simulink library "MISSILE_GUIDANCE_LIB2"  (R2025b)
settings: Solver=VariableStepAuto  StartTime=0.0  StopTime=10.0  RelTol=1e-3
undefined symbols (not defined in the file or in its folder): accelerationL0, angularPoseL0, angularRateL0, B2D, Continuous, ddLambda, dLambda, dRange, epsMEAS_D, L02B, Lambda, positionL0, psiDotCmd, psiMeas, Range, rangeDotMEAS_D, rangeMEAS_D, t_go, t_sim, targetEps_D, targetRelPos_B, targetRelPos_D, targetRelPos_L0, targetRelVel_L0, targetValid, thetaDotCmd, thetaMeas, Time, timeOfMeas, velocityL0, wAfterStabTF, wCmd_Rtn
libraries: $bdroot x27, simulink x8, simulink_extras x6, matrix_library x3, Missile_Guidance_LIB x1, ctrlSharedLib x1
(part 2 of 2)

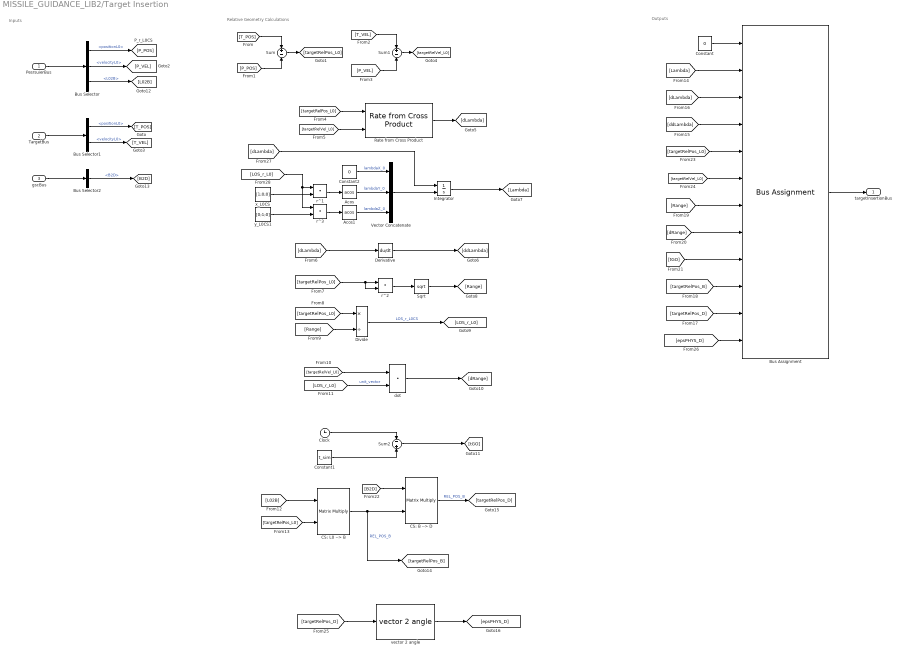
== system MISSILE_GUIDANCE_LIB2/Target Insertion ==
  note: Outputs
  note: Relative Geometry Calculations
  note: Inputs
  PesrsuierBus : Inport  OutDataTypeStr=Bus: missileBus
  TargetBus : Inport  Port=2  OutDataTypeStr=Bus: missileBus
  gscBus : Inport  Port=3  OutDataTypeStr=Bus: GscOutBus
  Acos : Trigonometry  Operator=acos
  Acos1 : Trigonometry  Operator=acos
  Bus Assignment : BusAssignment  AssignedSignals=Lambda,dLambda,ddLambda,targetRelPos_L0,targetRelVel_L0,Range,dRange,t_go,targetRelPos_B,targetRelPos_D,targetEps_D
  Bus Selector : BusSelector  OutputSignals=positionL0,velocityL0,L02B
  Bus Selector1 : BusSelector  OutputSignals=positionL0,velocityL0
  Bus Selector2 : BusSelector  OutputSignals=B2D
  CS: B --> D : Product  Multiplication=Matrix(*)
  CS: L0 --> B : Product  Multiplication=Matrix(*)
  Clock : Clock
  Constant : Constant  Value=0  OutDataTypeStr=Bus: targetInsertionBus
  Constant1 : Constant  Value=t_sim
  Constant2 : Constant  Value=0
  Derivative : Derivative
  Divide : Product  Inputs=*/
  Integrator : Integrator  InitialConditionSource=external
  Rate from Cross Product : $bdroot/Rate from Cross Product
  Sqrt : Sqrt
  Sum : Sum  Inputs=+|-
  Sum1 : Sum  Inputs=+|-
  Sum2 : Sum  Inputs=-|+
  Vector Concatenate : Concatenate  NumInputs=3
  dot : DotProduct  OutDataTypeStr=Inherit: Inherit via internal rule
  r^1 : DotProduct  OutDataTypeStr=Inherit: Inherit via internal rule
  r^2 : DotProduct  OutDataTypeStr=Inherit: Inherit via internal rule
  r^3 : DotProduct  OutDataTypeStr=Inherit: Inherit via internal rule
  vector 2 angle : $bdroot/vector 2 angle  SystemSampleTime=-1  VariantActivationTime=update diagram  AllowFlexibleInterface=on  Latency=0  AutoFrameSizeCalculation=off
  x_L0CS : Constant  Value=[1;0;0]
  y_L0CS1 : Constant  Value=[0;1;0]
  targetInsertionBus : Outport  OutDataTypeStr=Bus: targetInsertionBus
  wires:
  PesrsuierBus/1 -> Bus Selector/1
  Bus Selector/1 -> [P_POS]  "<positionL0>"
  TargetBus/1 -> Bus Selector1/1
  Bus Selector1/1 -> [T_POS]  "<positionL0>"
  Bus Selector1/2 -> [T_VEL]  "<velocityL0>"
  [T_POS] -> Sum/1
  [P_POS] -> Sum/2
  Sum/1 -> [targetRelPos_L0]
  Bus Selector/2 -> [P_VEL]  "<velocityL0>"
  [T_VEL] -> Sum1/1
  [P_VEL] -> Sum1/2
  Sum1/1 -> [targetRelVel_L0]
  [targetRelPos_L0] -> Rate from Cross Product/1
  [targetRelVel_L0] -> Rate from Cross Product/2
  Rate from Cross Product/1 -> [dLambda]
  [dLambda] -> Derivative/1
  Derivative/1 -> [ddLambda]
  Integrator/1 -> [Lambda]
  Constant/1 -> Bus Assignment/1
  Bus Assignment/1 -> targetInsertionBus/1
  r^2/1 -> Sqrt/1
  [targetRelPos_L0] -> r^2/2, r^2/1
  Sqrt/1 -> [Range]
  [targetRelPos_L0] -> Divide/1
  [Range] -> Divide/2
  Divide/1 -> [LOS_r_L0]  "LOS_r_L0CS"
  [targetRelVel_L0] -> dot/1
  [LOS_r_L0] -> dot/2  "unit_vector"
  Sum2/1 -> [tGO]
  [Lambda] -> Bus Assignment/2
  [dLambda] -> Bus Assignment/3
  [ddLambda] -> Bus Assignment/4
  [targetRelPos_L0] -> Bus Assignment/5
  [targetRelVel_L0] -> Bus Assignment/6
  [Range] -> Bus Assignment/7
  [dRange] -> Bus Assignment/8
  [tGO] -> Bus Assignment/9
  Clock/1 -> Sum2/1
  Constant1/1 -> Sum2/2
  Bus Selector/3 -> [L02B]  "<L02B>"
  gscBus/1 -> Bus Selector2/1
  Bus Selector2/1 -> [B2D]  "<B2D>"
  CS: L0 --> B/1 -> CS: B --> D/2, [targetRelPos_B]  "REL_POS_B"
  [L02B] -> CS: L0 --> B/1
  [targetRelPos_L0] -> CS: L0 --> B/2
  [B2D] -> CS: B --> D/1
  CS: B --> D/1 -> [targetRelPos_D]  "REL_POS_B"
  dot/1 -> [dRange]
  [targetRelPos_D] -> Bus Assignment/11
  [targetRelPos_B] -> Bus Assignment/10
  [targetRelPos_D] -> vector 2 angle/1
  vector 2 angle/1 -> [epsPHYS_D]
  [epsPHYS_D] -> Bus Assignment/12
  [LOS_r_L0] -> r^3/1, r^1/1
  x_L0CS/1 -> r^1/2
  r^1/1 -> Acos/1
  y_L0CS1/1 -> r^3/2
  Acos/1 -> Vector Concatenate/2  "lambdaY_0"
  r^3/1 -> Acos1/1
  Acos1/1 -> Vector Concatenate/3  "lambdaZ_0"
  [dLambda] -> Integrator/1
  Constant2/1 -> Vector Concatenate/1  "lambdaX_0"
  Vector Concatenate/1 -> Integrator/2

== system MISSILE_GUIDANCE_LIB2/TrueProNav ==
  Vc : Inport
  dotLambda : Inport  Port=2
  Constant : Constant  Value=N
  Product : Product  Inputs=3
  a_P_True : Outport
  wires:
  Constant/1 -> Product/1
  Product/1 -> a_P_True/1
  dotLambda/1 -> Product/3
  Vc/1 -> Product/2

== system MISSILE_GUIDANCE_LIB2/adding Scaled Noise ==
  pureSignal : Inport
  Product : Product
  Random Number : RandomNumber
  Sign : Signum
  Sum : Sum  Inputs=|++
  noise gain : Gain  Gain=noiseProc/100
  signalWithNoise : Outport
  wires:
  pureSignal/1 -> Sum/1, Product/1
  Random Number/1 -> Sign/1
  Product/1 -> noise gain/1
  Sign/1 -> Product/2
  Sum/1 -> signalWithNoise/1
  noise gain/1 -> Sum/2

== system MISSILE_GUIDANCE_LIB2/protected Division ==
  den : Inport
  num : Inport  Port=2
  Compare To Constant : simulink/Logic and Bit Operations/Compare To Constant  relop=~=  const=0  OutDataTypeStr=boolean
  Enabled Subsystem : Subsystem  TreatAsAtomicUnit=on
  res : Outport
  wires:
  den/1 -> Enabled Subsystem/2(den), Compare To Constant/1
  num/1 -> Enabled Subsystem/1(num)
  Enabled Subsystem/1(Result) -> res/1
  Compare To Constant/1 -> Enabled Subsystem/Enable

== system MISSILE_GUIDANCE_LIB2/rotateX ==
  phiAngle_RAD : Inport
  MATLAB Function : MATLAB Function  TreatAsAtomicUnit=on
  rotationMatrix : Outport
  wires:
  phiAngle_RAD/1 -> MATLAB Function/1(t)
  MATLAB Function/1(y) -> rotationMatrix/1

== system MISSILE_GUIDANCE_LIB2/rotateY ==
  thetaAngle_RAD : Inport
  MATLAB Function : MATLAB Function  TreatAsAtomicUnit=on
  rotationMatrix : Outport
  wires:
  thetaAngle_RAD/1 -> MATLAB Function/1(t)
  MATLAB Function/1(y) -> rotationMatrix/1

== system MISSILE_GUIDANCE_LIB2/rotateZ ==
  psiAngle_RAD : Inport
  MATLAB Function : MATLAB Function  TreatAsAtomicUnit=on
  rotationMatrix : Outport
  wires:
  MATLAB Function/1(y) -> rotationMatrix/1
  psiAngle_RAD/1 -> MATLAB Function/1(t)

== system MISSILE_GUIDANCE_LIB2/tGO_Estimator ==
  note: Output
  note: tGO Estimator
  note: Input
  targetInsertionBus : Inport  OutDataTypeStr=Bus: targetInsertionBus
  Bus Selector : BusSelector  OutputSignals=dRange,Range
  protected Division : $bdroot/protected Division  SystemSampleTime=-1  VariantActivationTime=update diagram  AllowFlexibleInterface=on  Latency=0  AutoFrameSizeCalculation=off
  tGO_Est : Outport
  wires:
  [dRange] -> protected Division/1
  protected Division/1 -> [tGO]
  [Range] -> protected Division/2
  targetInsertionBus/1 -> Bus Selector/1
  Bus Selector/1 -> [dRange]  "<dRange>"
  Bus Selector/2 -> [Range]  "<Range>"
  [tGO] -> tGO_Est/1

== system MISSILE_GUIDANCE_LIB2/vector 2 angle ==
  note: $\varepsilon_{VER} = atn2 \left( \frac{-R_z}{R_x} \right) \\\varepsilon_{HOR} = atn2 \left( \frac{R_y}{R_x} \right)$
  rX rY rZ : Inport
  Demux : Demux  Outputs=3
  Gain : Gain  Gain=-1
  Vector Concatenate : Concatenate  Mode=Multidimensional array
  epsHor : Trigonometry  Operator=atan2
  epsVer : Trigonometry  Operator=atan2
  epsVer epsHor : Outport
  wires:
  rX rY rZ/1 -> Demux/1
  epsVer/1 -> Vector Concatenate/1
  Vector Concatenate/1 -> [epsTarget_DCS]  "epsVer epsHor"
  [rX] -> epsHor/2
  [rY] -> epsHor/1
  epsHor/1 -> Vector Concatenate/2
  [rZ] -> Gain/1
  Gain/1 -> epsVer/1
  [rX] -> epsVer/2
  Demux/3 -> [rZ]
  Demux/1 -> [rX]
  Demux/2 -> [rY]
  [epsTarget_DCS] -> epsVer epsHor/1

== system MISSILE_GUIDANCE_LIB2/2D nonLinear Kinematics true ProNav/DCM_p2i ==
  note: $DCM = \left[ \matrix{C\lambda & -S\lambda \cr S\lambda & C\lambda} \right]$
  angle : Inport
  Cos : Trigonometry  Operator=cos
  Cos1 : Trigonometry
  Gain2 : Gain  Gain=-1
  Reshape : Reshape  OutputDimensionality=Customize  OutputDimensions=[2,2]
  Vector Concatenate : Concatenate  NumInputs=4
  DCM : Outport
  wires:
  Gain2/1 -> Vector Concatenate/3  "-S_angle"
  angle/1 -> Cos1/1, Cos/1
  Cos/1 -> Vector Concatenate/4, Vector Concatenate/1  "C_angle"
  Cos1/1 -> Vector Concatenate/2, Gain2/1  "S_angle"
  Vector Concatenate/1 -> Reshape/1
  Reshape/1 -> DCM/1

== system MISSILE_GUIDANCE_LIB2/2D nonLinear Kinematics true ProNav/DCM_t2i ==
  note: $DCM = \left[ \matrix{-C\beta & S\beta \cr S\beta & C\beta} \right]$
  angle : Inport
  Cos : Trigonometry  Operator=cos
  Cos1 : Trigonometry
  Gain : Gain  Gain=-1
  Reshape : Reshape  OutputDimensionality=Customize  OutputDimensions=[2,2]
  Vector Concatenate : Concatenate  NumInputs=4
  DCM : Outport
  wires:
  Reshape/1 -> DCM/1
  Vector Concatenate/1 -> Reshape/1
  Cos1/1 -> Vector Concatenate/2, Vector Concatenate/3  "S_angle"
  Gain/1 -> Vector Concatenate/1  "-C_angle"
  Cos/1 -> Gain/1, Vector Concatenate/4  "C_angle"
  angle/1 -> Cos/1, Cos1/1

== system MISSILE_GUIDANCE_LIB2/Simple GSC/If Action Subsystem ==
  B2D : Inport
  Action Port : ActionPort  ActionPortLabel=case [ 1 ]:
  Out1 : Outport
  wires:
  B2D/1 -> Out1/1

== system MISSILE_GUIDANCE_LIB2/Simple GSC/If Action Subsystem1 ==
  B2D : Inport
  Action Port : ActionPort  ActionPortLabel=case [ 0 ]:
  Out1 : Outport
  wires:
  B2D/1 -> Out1/1

== system MISSILE_GUIDANCE_LIB2/Simple GSC/RATE TF ==
  In1 : Inport
  Demux : Demux  Outputs=3
  TF RATE : TransferFcn  Numerator=(2*pi*fRATE)^2  Denominator=[1 2*zetaRATE*(2*pi*fRATE) (2*pi*fRATE)^2]
  TF RATE1 : TransferFcn  Numerator=(2*pi*fRATE)^2  Denominator=[1 2*zetaRATE*(2*pi*fRATE) (2*pi*fRATE)^2]
  TF RATE2 : TransferFcn  Numerator=(2*pi*fRATE)^2  Denominator=[1 2*zetaRATE*(2*pi*fRATE) (2*pi*fRATE)^2]
  Vector Concatenate : Concatenate  NumInputs=3  Mode=Multidimensional array
  Out1 : Outport
  wires:
  In1/1 -> Demux/1
  Demux/2 -> TF RATE/1  "wVerCmd"
  Demux/1 -> TF RATE1/1  "wX"
  Demux/3 -> TF RATE2/1  "wHorCmd"
  TF RATE/1 -> Vector Concatenate/2
  TF RATE2/1 -> Vector Concatenate/3
  TF RATE1/1 -> Vector Concatenate/1
  Vector Concatenate/1 -> Out1/1

== system MISSILE_GUIDANCE_LIB2/Simple LOS/Enabled Subsystem ==
  In1 : Inport
  Action Port : ActionPort  ActionPortLabel=case [ 1 ]:
  Out1 : Outport
  wires:
  In1/1 -> Out1/1

== system MISSILE_GUIDANCE_LIB2/Simple LOS/Enabled Subsystem1 ==
  In1 : Inport
  Action Port : ActionPort  ActionPortLabel=case [ 0 ]:
  Out1 : Outport
  wires:
  In1/1 -> Out1/1

== system MISSILE_GUIDANCE_LIB2/SimpleSensor/Range Measurements ==
  PHYS : Inport
  Enable : EnablePort
  MEAS : Outport  OutputWhenDisabled=reset  InitialOutput=0
  wires:
  PHYS/1 -> MEAS/1

== system MISSILE_GUIDANCE_LIB2/SimpleSensor/Rnge Dot Measurements ==
  PHYS : Inport
  Enable : EnablePort
  MEAS : Outport  OutputWhenDisabled=reset  InitialOutput=[0]
  wires:
  PHYS/1 -> MEAS/1

== system MISSILE_GUIDANCE_LIB2/SimpleSensor/epsilon Measurements ==
  PHYS : Inport
  Enable : EnablePort
  MEAS : Outport  OutputWhenDisabled=reset  InitialOutput=[0;0]
  wires:
  PHYS/1 -> MEAS/1

== system MISSILE_GUIDANCE_LIB2/protected Division/Enabled Subsystem ==
  num : Inport
  den : Inport  Port=2
  Enable : EnablePort
  Divide : Product  Inputs=*/
  Result : Outport  OutputWhenDisabled=reset  InitialOutput=[0]
  wires:
  num/1 -> Divide/1
  den/1 -> Divide/2
  Divide/1 -> Result/1

== matlab function MISSILE_GUIDANCE_LIB2/Direct Integration of Euler KDE/MATLAB Function ==
  data: posVec input; A output
function  A = fcn(posVec)

phi = posVec(3);
theta = posVec(2);
psi = posVec(1);


MAT = [    0              sin(phi)                cos(phi);...
         0          cos(phi)*cos(theta)     -sin(phi)*cos(theta);...
     cos(theta)    sin(phi)*sin(theta)      cos(phi)*sin(theta)];


A =1/cos(theta)*MAT;
end

== matlab function MISSILE_GUIDANCE_LIB2/LOS ESTIMATOR/A matrix ==
  data: Wlos input; A output
function A = fcn(Wlos)

Wx = Wlos(1);

A = zeros(6,6);

A(1,2) = 1;
A(1,4) = Wx;

A(2,3) = 1;
A(2,5) = Wx;

A(4,1) = (-1)*Wx;
A(4,5) = 1;

A(5,2) = (-1)*Wx;
A(5,6) = 1;

== matlab function MISSILE_GUIDANCE_LIB2/LOS ESTIMATOR/B matrix ==
  data: B output
function B = fcn()

B = zeros(6,2);

B(1,1) = (-1);
B(4,2) = (-1);

== matlab function MISSILE_GUIDANCE_LIB2/LOS ESTIMATOR/C matrix ==
  data: C output
function C = fcn()

C = zeros(2,6);

C(1,1) = 1;
C(2,4) = 1;

== matlab function MISSILE_GUIDANCE_LIB2/Animation 3D ==
  settings: updateMethod=DISCRETE
  data: R_T input; R_P input
function fcn(R_T, R_P)

R_Tx = R_T(1,1);
R_Ty = R_T(2,1);
R_Tz = R_T(3,1);

R_Px = R_P(1,1);
R_Py = R_P(2,1);
R_Pz = R_P(3,1);


plot3(R_Tx, R_Ty, R_Tz, 'r.-', 'MarkerSize', 15); hold on
plot3(R_Px, R_Py, R_Pz, 'b.-', 'MarkerSize',15)


drawnow

end

== matlab function MISSILE_GUIDANCE_LIB2/rotateX/MATLAB Function ==
  data: t input; y output
function y = rotx(t)

y = [1    0       0; 
             0   cos(t) sin(t); 
             0   -sin(t)  cos(t)];

== matlab function MISSILE_GUIDANCE_LIB2/rotateY/MATLAB Function ==
  data: t input; y output
function y = roty(t)

y = [cos(t)   0   -sin(t); 
              0       1    0 ;
            sin(t)   0   cos(t)];

== matlab function MISSILE_GUIDANCE_LIB2/rotateZ/MATLAB Function ==
  data: t input; y output
function y = rotz(t)

y = [cos(t)  sin(t)   0 ; 
   -sin(t)   cos(t)   0 ; 
     0        0       1];

== matlab function MISSILE_GUIDANCE_LIB2/Euler2DCM/eul2rotm ==
  data: u input; y output
function y = fcn(u)

y = eul2rotm(u');

== matlab function MISSILE_GUIDANCE_LIB2/LOS ESTIMATOR/D matrix ==
  data: D output
function D = fcn()

D = zeros(2,2);

== matlab function MISSILE_GUIDANCE_LIB2/Animation 2D ==
  settings: updateMethod=DISCRETE
  data: R_T input; R_P input
function fcn(R_T, R_P)

R_Tx = R_T(1);
R_Tz = R_T(2);
R_Px = R_P(1);
R_Pz = R_P(2);


plot(R_Tx, R_Tz, 'r.-', 'MarkerSize', 15); hold on
plot(R_Px, R_Pz, 'b.-', 'MarkerSize',15)


drawnow

end
